simulink model "plasticWelderSim"  (R2015b)
settings: Solver=VariableStepAuto  StartTime=0.0  StopTime=1200  RelTol=1e-3
libraries: simulink x1
settings Model: Creator=Derek  LastModifiedBy=Derek

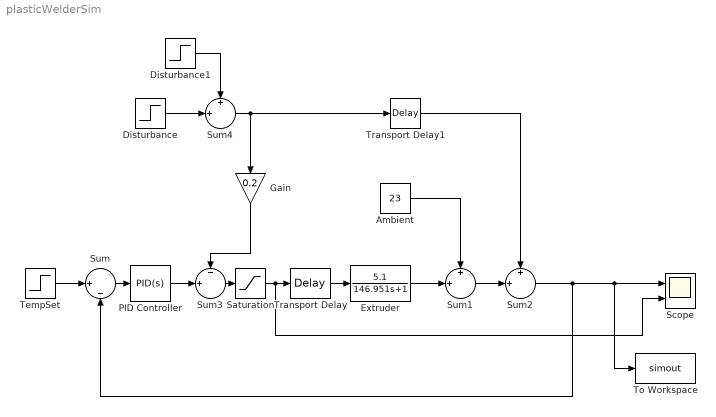
== system plasticWelderSim ==
  Ambient : Constant  Value=23
  Disturbance : Step  Time=700  After=-10  SampleTime=0
  Disturbance1 : Step  Time=800  After=10  SampleTime=0
  Extruder : TransferFcn  Numerator=[5.1]  Denominator=[146.951 1]
  Gain : Gain  Gain=0.2
  PID Controller : simulink/Continuous/PID Controller  Controller=PID  TimeDomain=Continuous-time  SampleTime=-1  IntegratorMethod=Forward Euler  FilterMethod=Forward Euler  Form=Parallel  UseFilter=on  ControllerParametersSource=internal  P=1.48134292984995  I=0.0131800567660014  D=18.6947422906608  N=0.169991587444944  InitialConditionSource=internal  InitialConditionForIntegrator=0  InitialConditionForFilter=0  ExternalReset=none  LimitOutput=on  UpperSaturationLimit=100  LowerSaturationLimit=0  LinearizeAsGain=on  AntiWindupMode=clamping  Kb=1  TrackingMode=off  Kt=1  PParamMin=[]  PParamMax=[]  IParamMin=[]  IParamMax=[]  DParamMin=[]  DParamMax=[]  NParamMin=[]  NParamMax=[]  KbParamMin=[]  KbParamMax=[]  KtParamMin=[]  KtParamMax=[]  POutMin=[]  POutMax=[]  IOutMin=[]  IOutMax=[]  DOutMin=[]  DOutMax=[]  NOutMin=[]  NOutMax=[]  KbOutMin=[]  KbOutMax=[]  KtOutMin=[]  KtOutMax=[]  IntegratorOutMin=[]  IntegratorOutMax=[]  FilterOutMin=[]  FilterOutMax=[]  SumOutMin=[]  SumOutMax=[]  SumI1OutMin=[]  SumI1OutMax=[]  SumI2OutMin=[]  SumI2OutMax=[]  SumI3OutMin=[]  SumI3OutMax=[]  SumDOutMin=[]  SumDOutMax=[]  SaturationOutMin=[]  SaturationOutMax=[]  IntegratorContinuousStateAttributes=''  IntegratorStateMustResolveToSignalObject=off  IntegratorRTWStateStorageClass=Auto  FilterContinuousStateAttributes=''  FilterStateMustResolveToSignalObject=off  FilterRTWStateStorageClass=Auto  DifferentiatorICPrevScaledInput=0  DifferentiatorOutMin=[]  DifferentiatorOutMax=[]
  Saturation : Saturate  UpperLimit=100  LowerLimit=0
  Scope : Scope  NumInputPorts=2
  Sum : Sum  Inputs=||+|-
  Sum1 : Sum  Inputs=+|+||
  Sum2 : Sum  Inputs=+|+||
  Sum3 : Sum  Inputs=-|+||
  Sum4 : Sum  Inputs=+|+||
  "TempSet " : Step  Time=200  After=100  SampleTime=.5
  To Workspace : ToWorkspace  VariableName=simout  SampleTime=.5
      settings: MaxDataPoints=1800  Save2DSignal=2-D array (concatenate along first dimension)
  Transport Delay : TransportDelay  DelayTime=7
  Transport Delay1 : TransportDelay  DelayTime=5
  wires:
  "TempSet "/1 -> Sum/1
  Ambient/1 -> Sum1/1
  Extruder/1 -> Sum1/2
  Transport Delay/1 -> Extruder/1
  Sum1/1 -> Sum2/2
  Sum/1 -> PID Controller/1
  Saturation/1 -> Scope/2, Transport Delay/1
  Sum2/1 -> Sum/2, To Workspace/1, Scope/1
  Transport Delay1/1 -> Sum2/1
  PID Controller/1 -> Sum3/2
  Sum3/1 -> Saturation/1
  Sum4/1 -> Gain/1, Transport Delay1/1
  Disturbance/1 -> Sum4/2
  Disturbance1/1 -> Sum4/1
  Gain/1 -> Sum3/1
